simulink model "simul_task2"  (R2021b)
settings: Solver=FixedStepAuto  StartTime=0.0  StopTime=10.0  FixedStep=10e-5  RelTol=1e-3
undefined symbols (not defined in the file): A, B, C, D, F, I
settings Model: Creator=witold  LastModifiedBy=witold

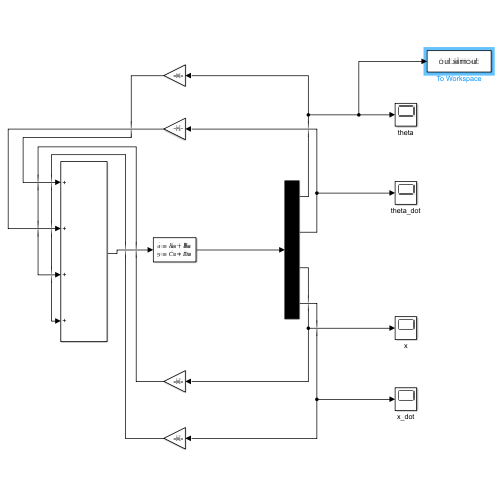
[thumbnail: Simulink's stored preview of the top-level diagram]
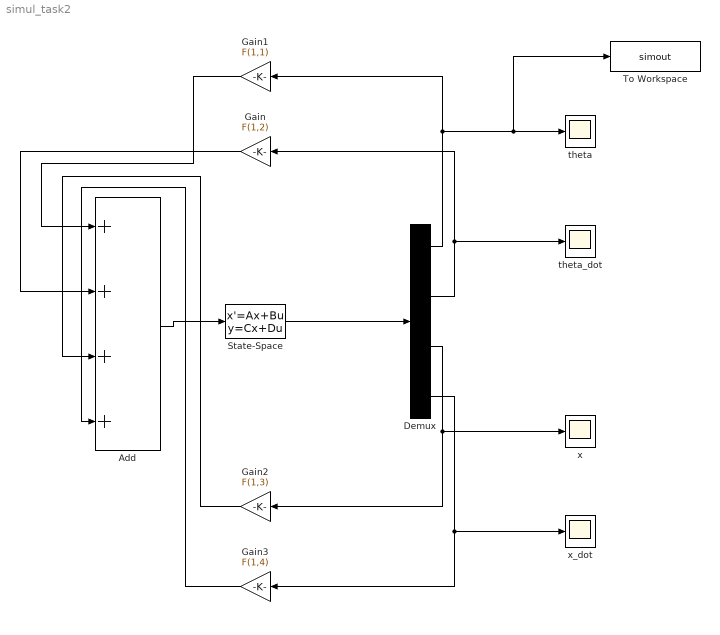
== system simul_task2 ==
  Add : Sum  Inputs=++++
  Demux : Demux
  Gain : Gain  Gain=F(1,2)
  Gain1 : Gain  Gain=F(1,1)
  Gain2 : Gain  Gain=F(1,3)
  Gain3 : Gain  Gain=F(1,4)
  State-Space : StateSpace  A=A  B=B  C=C  D=D  InitialCondition=I  ContinuousStateAttributes={'th' , 'thdot', 'x', 'xdot'}
  To Workspace : ToWorkspace  VariableName=simout  SampleTime=-1
  theta : Scope
  theta_dot : Scope
  x : Scope
  x_dot : Scope
  wires:
  State-Space/1 -> Demux/1
  Add/1 -> State-Space/1
  Demux/3 -> Gain2/1, x/1
  Demux/4 -> Gain3/1, x_dot/1
  Gain2/1 -> Add/3
  Gain3/1 -> Add/4
  Gain/1 -> Add/2
  Gain1/1 -> Add/1
  Demux/2 -> theta_dot/1, Gain/1
  Demux/1 -> Gain1/1, To Workspace/1, theta/1
